simulink model "simulink_Test"  (R2016b)
settings: Solver=VariableStepAuto  StartTime=0.0  StopTime=10.0  RelTol=1e-3
settings Model: Creator=ga69qig  LastModifiedBy=ga69qig

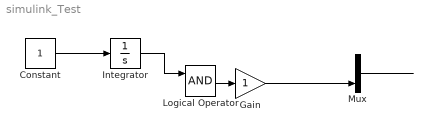
== system simulink_Test ==
  Constant : Constant
  Gain : Gain
  Integrator : Integrator
  Logical Operator : Logic  AllPortsSameDT=off  OutDataTypeStr=boolean
  Mux : Mux  Inputs=2
  wires:
  Mux/1 -> ?
  Constant/1 -> Integrator/1
  Integrator/1 -> Logical Operator/1
  Logical Operator/1 -> Gain/1
  Gain/1 -> Mux/2
